simulink model "Ex2_4"  (R2016a)
settings: Solver=VariableStepAuto  StartTime=0.0  StopTime=10.0  RelTol=1e-3
settings Model: Creator=mende  LastModifiedBy=mende

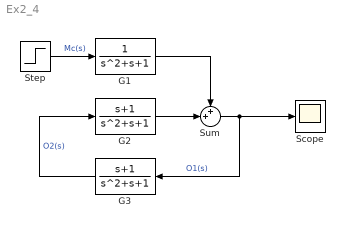
== system Ex2_4 ==
  G1 : TransferFcn  Denominator=[1 1 1]
  G2 : TransferFcn  Numerator=[1 1]  Denominator=[1 1 1]
  G3 : TransferFcn  Numerator=[1 1]  Denominator=[1 1 1]
  Scope : Scope
  Step : Step  SampleTime=0
  Sum : Sum  Inputs=++|
  wires:
  Sum/1 -> G3/1, Scope/1  "O1(s)"
  G1/1 -> Sum/1
  G2/1 -> Sum/2
  G3/1 -> G2/1  "O2(s)"
  Step/1 -> G1/1  "Mc(s)"
